simulink model "FullTrackTableModel_Annotated"  (R2020b)
settings: Solver=VariableStepAuto  StartTime=0.0  StopTime=10.0  RelTol=1e-3
undefined symbols (not defined in the file): sigbuilder_block
settings Model: Creator=joems  LastModifiedBy=joems

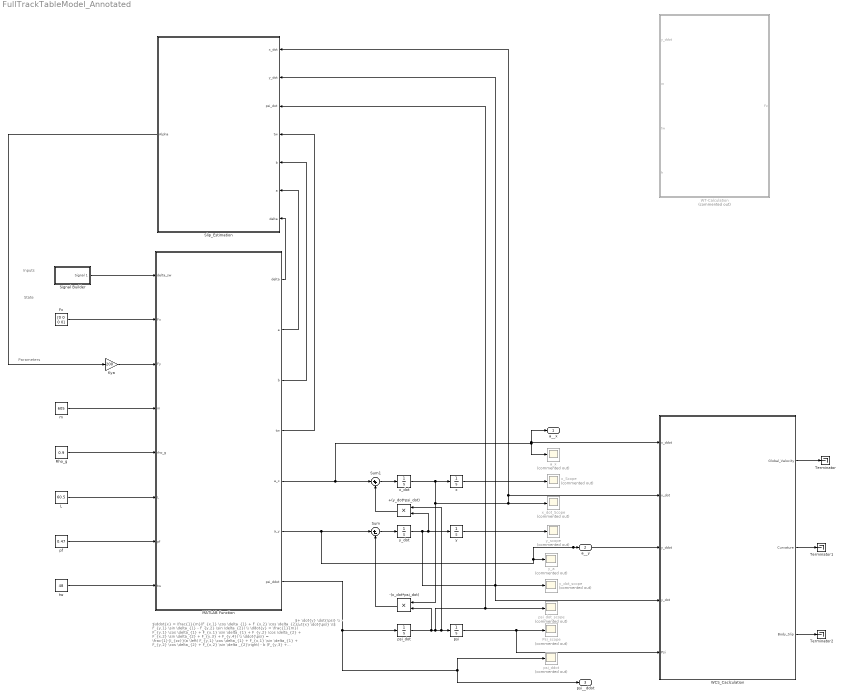
== system FullTrackTableModel_Annotated ==
  note: $+ \dot{y} \dot{\psi} \\ - \dot{x} \dot{\psi} \\$
  note: $\ddot{x} = \frac{1}{m}(F_{x,1} \cos \delta_{1} + F_{x,2} \cos \delta_{2} - F_{y,1} \sin \delta_{1} - F_{y,2} \sin \delta_{2}) \\ \ddot{y} = \frac{1}{m}( F_{y,1} \cos \delta_{1} + F_{x,1} \sin \delta_{1} + F_{y,2} \cos \delta_{2} + F_{x,2} \sin \delta_{2} + F_{y,3} + F_{y,4}) \\ \ddot{\psi} = \frac{1}{I_{zz}}(a \left( F_{y,1} \cos \delta_{1} + F_{x,1} \sin \delta_{1} + F_{y,2} \cos \delta_{2} + F_{x,2} \sin \delta _{2}\right) - b (F_{y,3} + F_{y,4}))$
  note: State
  note: Inputs
  note: Parameters
  +(y_dot*psi_dot) : Product
  -(x_dot*psi_dot) : Product
  Fx : Constant  Value=[0 0 0 0]
  Kya : Gain  Gain=200
  L : Constant  Value=60.5
  MATLAB Function : MATLAB Function  TreatAsAtomicUnit=on
  Psi_scope : Scope  Commented=on
  Rho_g : Constant  Value=0.9
  Signal Builder : Subsystem  Tag=STV Subsys  LoadFcn=sigbuilder_block('load',[437.6 199.2 550.4 400 ]);  StartFcn=sigbuilder_block('start');  StopFcn=sigbuilder_block('stop');  ClipboardFcn=sigbuilder_block('clipboard');  mask(Sigbuilder block){tuvar=[0:10]}
      mask help: Simulink:masks:SigbuilderBlock_MD
      mask init:
      | if ~strcmp(get_param(bdroot(gcbh),'SimulationStatus'),'stopped') tuvar = sigbuilder_block('maskInit'); end
      settings: CopyFcn=sigbuilder_block('copy');  DeleteFcn=sigbuilder_block('delete');  ModelCloseFcn=sigbuilder_block('modelClose');  PreSaveFcn=sigbuilder_block('preSave');  PauseFcn=sigbuilder_block('pause');  ContinueFcn=sigbuilder_block('continue');  NameChangeFcn=sigbuilder_block('namechange');  OpenFcn=sigbuilder_block('open',[437.6 199.2 550.4 400 ]);  CloseFcn=sigbuilder_block('close');
      mask Display: plot(0, 0, 100, 100,[2, 2, 32, 32, 2], [68, 8, 8, 68, 68],[32, 2], [38, 38], [32, 19, 2],[53, 60, 44], [32, 17, 17, 2],[16, 16, 31, 31]);txt = getActiveGroup(gcbh);text(2, 100, txt,'verticalAlignment', 'top');
  Slip_Estimation : MATLAB Function  TreatAsAtomicUnit=on
  Sum : Sum  Inputs=|+-
  Sum1 : Sum  Inputs=|++
  Terminator : Terminator
  Terminator1 : Terminator
  Terminator2 : Terminator
  "WCS_Caclculation " : MATLAB Function  TreatAsAtomicUnit=on
  WT-Calculation : MATLAB Function  Commented=on  TreatAsAtomicUnit=on
  a_x : Scope  Commented=on
  m : Constant  Value=605
  pf : Constant  Value=0.47
  psi : Integrator
  psi_ddot : Scope  Commented=on
  psi_dot : Integrator
  psi_dot_scope : Scope  Commented=on
  tw : Constant  Value=48
  x : Integrator
  x_Scope : Scope  Commented=on
  x_dot : Integrator  InitialCondition=30
  x_dot_Scope : Scope  Commented=on
  y : Integrator
  y_a : Scope  Commented=on
  y_dot : Integrator
  y_dot_scope : Scope  Commented=on
  y_scope : Scope  Commented=on
  a__x : Outport
  a__y : Outport  Port=2
  psi__ddot : Outport  Port=3
  wires:
  Fx/1 -> MATLAB Function/2(Fx)
  m/1 -> MATLAB Function/4(m)
  Rho_g/1 -> MATLAB Function/5(rho_g)
  L/1 -> MATLAB Function/6(L)
  pf/1 -> MATLAB Function/7(pf)
  MATLAB Function/6(a_y) -> Sum/1, "WCS_Caclculation "/3(y_ddot), a__y/1, y_a/1
  -(x_dot*psi_dot)/1 -> Sum/2
  +(y_dot*psi_dot)/1 -> Sum1/2
  MATLAB Function/5(a_x) -> Sum1/1, a__x/1, "WCS_Caclculation "/1(x_ddot), a_x/1
  Sum1/1 -> x_dot/1
  Sum/1 -> y_dot/1
  y_dot/1 -> Slip_Estimation/2(y_dot), "WCS_Caclculation "/4(y_dot), y_dot_scope/1, y/1, +(y_dot*psi_dot)/2
  psi/1 -> "WCS_Caclculation "/5(Psi), Psi_scope/1
  y/1 -> y_scope/1
  x/1 -> x_Scope/1
  MATLAB Function/7(psi_ddot) -> psi_dot/1, psi__ddot/1, psi_ddot/1
  tw/1 -> MATLAB Function/8("tw ")
  MATLAB Function/2(a) -> Slip_Estimation/6(a)
  MATLAB Function/3(b) -> Slip_Estimation/5(b)
  MATLAB Function/4(tw) -> Slip_Estimation/4(tw)
  psi_dot/1 -> Slip_Estimation/3(psi_dot), psi_dot_scope/1, +(y_dot*psi_dot)/1, psi/1, -(x_dot*psi_dot)/2
  x_dot/1 -> "WCS_Caclculation "/2(x_dot), Slip_Estimation/1(x_dot), x_dot_Scope/1, -(x_dot*psi_dot)/1, x/1
  MATLAB Function/1(delta) -> Slip_Estimation/7(delta)
  "WCS_Caclculation "/1(Global_Velocity) -> Terminator/1
  "WCS_Caclculation "/3(Body_Slip) -> Terminator2/1
  "WCS_Caclculation "/2(Curvature) -> Terminator1/1
  Kya/1 -> MATLAB Function/3(Fy)
  Slip_Estimation/1(Alpha) -> Kya/1
  Signal Builder/1(Signal 1) -> MATLAB Function/1(delta_sw)

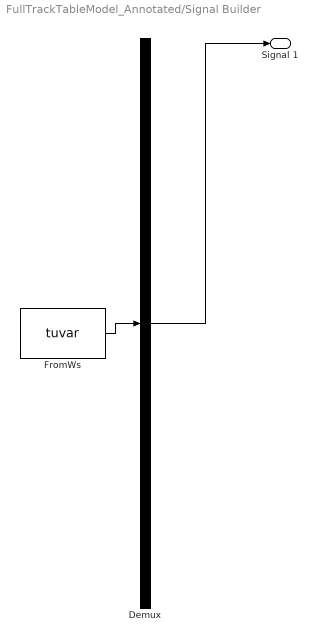
== system FullTrackTableModel_Annotated/Signal Builder ==
  Demux : Demux  Tag=STV Demux  Outputs=1
      settings: DisplayOption=none
  FromWs : FromWorkspace  Tag=STV FromWs  VariableName=tuvar
      SigBuilderData=|
      | common.afterFinalStr = 'Extrapolate'
      | common.sampleTime = 0
      | dataSet.timeRange = [0 10]
      | dataSet.name = 'Group 1'
      | sbobj.Groups.Name = 'Group 1'
      | sbobj.Groups.Signals.Name = 'Signal 1'
      | sbobj.Groups.Signals.XData = [0 4 4.3 10]
      | sbobj.Groups.Signals.YData = [0 0 10.05 10]
  Signal 1 : Outport  Tag=STV Outport
  wires:
  Demux/1 -> Signal 1/1
  FromWs/1 -> Demux/1

== matlab function FullTrackTableModel_Annotated/Slip_Estimation ==
  data: x_dot input; y_dot input; psi_dot input; tw input; b input; a input; delta input; Alpha output
function Alpha = Slip_Estimation(x_dot, y_dot, psi_dot, tw, b, a, delta)

Alpha = zeros(1,4);

Alpha(1) = delta - atan2d( (y_dot + a.*psi_dot) ./ ( x_dot + ... 
    ( (tw/2).*psi_dot ) ), x_dot);

Alpha(2) = delta - atan2d( (y_dot + a.*psi_dot) ./ ( x_dot - ...
    ( (tw/2).*psi_dot ) ), x_dot);

Alpha(3) = - atan2d( (y_dot - b.*psi_dot)./ (x_dot + ...
    ( (tw/2).*psi_dot) ), x_dot);                                            %Note: there is no delta because the back wheels dont get steered 

Alpha(4) = - atan2d( (y_dot - b.*psi_dot) ./ (x_dot - ...
    ( (tw/2).*psi_dot) ) , x_dot);
end

== matlab function FullTrackTableModel_Annotated/MATLAB Function ==
  data: delta output; a output; b output; tw output; delta_sw input; Fx input size=[ 1 4 ]; a_x output; Fy input size=[ 1 4 ]; m input; rho_g input; L input; pf input; a_y output; psi_ddot output; tw input
function [delta, a, b, tw, a_x, a_y, psi_ddot]   = ...
    Acceleration_Function(delta_sw,Fx,Fy,m,rho_g,L,pf,tw)
%% Parameters 
tw = tw/39.3700787;
L = L/39.3700787;  
m = m/2.20462262;     %Conversions
a = L * (1 - pf);     %Because the ceneter or mass is more to there rear so a is longer
b = L * pf;
Izz = m * (rho_g)^2;  %Cacls
delta = 0.25 * delta_sw;  %Steering angle ratio to the rear steergin angle 

%% Logitudinal

a_x = ( Fx(1).*cosd(delta) + Fx(2).*cosd(delta) - ... 
        Fy(1).*sind(delta) - Fy(2).*sind(delta) + Fx(3) + Fx(4) ) / m; 
%% Lateral

a_y = ( Fy(1).*cosd(delta) + Fx(1).*sind(delta) + ...
        Fy(2).*cosd(delta) + Fx(2).*sind(delta) + Fy(3) + Fy(4) ) / m;

%% Yaw

psi_ddot = a.*( Fy(1) + Fy(2) ) - b.*( Fy(3) + Fy(4) ) + ...
           (tw/2).*( Fx(2) + Fx(4) ) - (tw/2).*( Fx(1) + Fx(3) )/Izz;
end

== matlab function FullTrackTableModel_Annotated/WCS_Caclculation  ==
  data: x_ddot input; x_dot input; y_ddot input; y_dot input; Psi input; Global_Velocity output; Curvature output; Body_Slip output
function [Global_Velocity, Curvature, Body_Slip] = ...
    WCS_Calculations( x_ddot, x_dot, y_ddot, y_dot, Psi)
%% Nomenclature
% Yaw Angle                : Psi
% Longitudinal Velocity    : x_dot
% Longitudinal Acceleration: x_ddot
% Lateral Velocity         : y_dot
% Lateral Acceleration     : y_ddot 

%% Global Displacement 
Global_Velocity = zeros(1,2);

Global_Velocity(1) = x_dot.*cosd(Psi) - y_dot.*sind(Psi);

Global_Velocity(2) =  x_dot.*sind(Psi) + y_dot.*cosd(Psi);

%% Curvature 
if abs( x_dot.^2 + y_dot.^2 ) <= 0.1;
    Curvature = 100;  
else 
    Curvature = abs( x_ddot.*y_dot - y_ddot.*x_dot )./ ...
        ( x_dot.^2 + y_dot.^2 ).^(3/2);
end 

%% Body Slip 

Body_Slip = atan2d(y_dot, x_dot);

end

== matlab function FullTrackTableModel_Annotated/WT-Calculation ==
  data: y_ddot input; Fz output; m input; tw input; h input
function Fz = WT_Calculation(y_ddot, m, tw, h) 

g = 9.81

Fz = zeros(1,2) %is this a 1 x4 or 1 x 2? I.E. are the front and back of the inner and outer equal?(In reality no, but in model?)

if y_ddot = 0 
    Fz(1) = 0.5*m*g
    Fz(2) = Fz(1) 
else 
    Fy = m*ay
    Fz(1) = 0.5*m*g - Fy*( h/tw ) 
    Fz(2) = Fz(1) + Fy*( ( 2*h/tw ) ) 
end 
end
